simulink model "loberotator_final"  (R2018a)
settings: Solver=VariableStepAuto  StartTime=0.0  StopTime=100  RelTol=1e-3
libraries: xbsIndex_r4 x104, xps_library x4, casper_library_misc x1
(part 2 of 4)

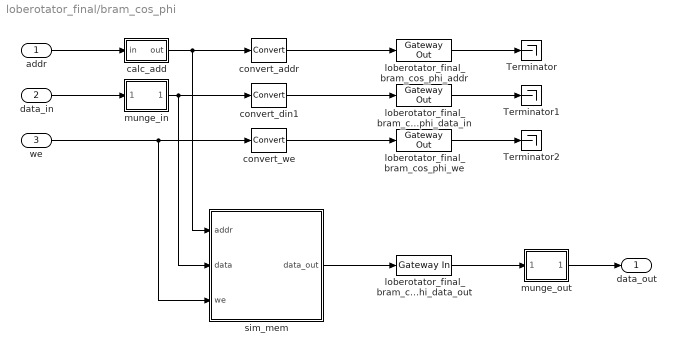
== system loberotator_final/bram_cos_phi ==
  addr : Inport
  data_in : Inport  Port=2
  we : Inport  Port=3
  Terminator : Terminator
  Terminator1 : Terminator
  Terminator2 : Terminator
  calc_add : Subsystem  mask{data_width=32, addr_width=11, sample_rate=sample_rate}
      mask prompts: data_width "data width"; addr_width "address width"; sample_rate "sample rate"
  convert_addr : xbsIndex_r4/Convert  gui_display_data_type=Fixed-point  arith_type=Unsigned  n_bits=addr_width  bin_pt=0  float_type=Single  exp_bits=8  fraction_bits=24  quantization=Truncate  overflow=Wrap  en=off  latency=0  pipeline=off  dbl_ovrd=off  block_type=convert
      settings: xl_area=[0, 0, 0, 0, 0, 0, 0]
  convert_din1 : xbsIndex_r4/Convert  gui_display_data_type=Fixed-point  arith_type=Unsigned  n_bits=32  bin_pt=0  float_type=Single  exp_bits=8  fraction_bits=24  quantization=Truncate  overflow=Wrap  en=off  latency=0  pipeline=off  dbl_ovrd=off  block_type=convert
      settings: xl_area=[0, 0, 0, 0, 0, 0, 0]
  convert_we : xbsIndex_r4/Convert  gui_display_data_type=Fixed-point  arith_type=Unsigned  n_bits=1  bin_pt=0  float_type=Single  exp_bits=8  fraction_bits=24  quantization=Truncate  overflow=Wrap  en=off  latency=0  pipeline=off  dbl_ovrd=off  block_type=convert
      settings: xl_area=[0, 0, 0, 0, 0, 0, 0]
  loberotator_final_bram_cos_phi_addr : xbsIndex_r4/Gateway Out  inherit_from_input=off  hdl_port=on  rows=1  columns=1  UseAsDAC=off  DACChannel='1'  interface=None  automatic_assignment=on  address_offset=hex2dec('00')  intf_name=''  intf_description=''  timing_constraint=None  locs_specified=off  LOCs={'A5','B9','A9','C1','A3','G6','E9','A6','A7','A8','B8','B1','B3','D9','B5','B4','B6','C2'}  io_standard={}  block_type=gatewayout
      settings: infoedit="Gateway out block.  Converts Xilinx fixed point inputs into ouputs of type Simulink integer, double, or fixed point.<P><P>Hardware notes:  In hardware these blocks become top level output ports or are discarded, depending on how they are configured."  sginterface={'Nallatech'=>{'xdspkit'=>{'non_memory_mapped_port'=>'uprev_Shared_BRAM_addr'}},'Xilinx'=>{'jtaghwcosim'=>{'non_memory_mapped_port'=>'uprev_Shared_BRAM_addr'},'xdspkit'=>{'non_memory_mapped_port'=>'uprev_Shared_BRAM_addr'}}}  xl_area=[0, 0, 0, 0, 0, 0, 0]
  loberotator_final_bram_cos_phi_data_in : xbsIndex_r4/Gateway Out  inherit_from_input=off  hdl_port=on  rows=1  columns=1  UseAsDAC=off  DACChannel='1'  interface=None  automatic_assignment=on  address_offset=hex2dec('00')  intf_name=''  intf_description=''  timing_constraint=None  locs_specified=off  LOCs={'B21','B22','A22','B23','B19','C19','A20','A21','A23','B24','A24','A25','E18','D18','C18','B18'}  io_standard={}  block_type=gatewayout
      settings: infoedit="Gateway out block.  Converts Xilinx fixed point inputs into ouputs of type Simulink integer, double, or fixed point.<P><P>Hardware notes:  In hardware these blocks become top level output ports or are discarded, depending on how they are configured."  sginterface={'Nallatech'=>{'xdspkit'=>{'non_memory_mapped_port'=>'uprev_Shared_BRAM_data_in'}},'Xilinx'=>{'jtaghwcosim'=>{'non_memory_mapped_port'=>'uprev_Shared_BRAM_data_in'},'xdspkit'=>{'non_memory_mapped_port'=>'uprev_Shared_BRAM_data_in'}}}  xl_area=[0, 0, 0, 0, 0, 0, 0]
  loberotator_final_bram_cos_phi_data_out : xbsIndex_r4/Gateway In  gui_display_data_type=Fixed-point  arith_type=Unsigned  n_bits=32  bin_pt=0  preci_type=Single  exp_width=8  frac_width=24  rows=1  columns=1  quantization=Truncate  overflow=Wrap  period=sample_rate  UseAsADC=off  ADCChannel='1'  interface=None  automatic_assignment=on  address_offset=hex2dec('00')  intf_name=''  intf_description=''  default_value=0  timing_constraint=None  locs_specified=off  LOCs={}  io_standard={}  inherit_from_input=off  hdl_port=on  dbl_ovrd=off  block_type=gatewayin
      settings: xl_area=[0, 0, 0, 0, 0, 0, 0]
  loberotator_final_bram_cos_phi_we : xbsIndex_r4/Gateway Out  inherit_from_input=off  hdl_port=on  rows=1  columns=1  UseAsDAC=off  DACChannel='1'  interface=None  automatic_assignment=on  address_offset=hex2dec('00')  intf_name=''  intf_description=''  timing_constraint=None  locs_specified=off  LOCs={'A14'}  io_standard={}  block_type=gatewayout
      settings: infoedit="Gateway out block.  Converts Xilinx fixed point inputs into ouputs of type Simulink integer, double, or fixed point.<P><P>Hardware notes:  In hardware these blocks become top level output ports or are discarded, depending on how they are configured."  xl_area=[0, 0, 0, 0, 0, 0, 0]
  munge_in : Subsystem  AncestorBlock=casper_library_flow_control/munge  mask(munge){divisions=1, div_size=32, order=[0], arith_type_out=Unsigned, bin_pt_out=0}
      mask prompts: divisions "Number of divisions"; div_size "Division size (bits)"; order "Division packing order"; arith_type_out "Output arithmetic type"; bin_pt_out "Output binary point"
      mask help: Splits an input bus into the specified number of divisions and then recombines them in the order specified (most significant division = 0,least = number divisions-1)
      mask init:
      | munge_init(gcb, ...
      |     'divisions', divisions, ...
      |     'div_size', div_size, ...
      |     'order', order, ...
      |     'arith_type_out', arith_type_out, ...
      |     'bin_pt_out', bin_pt_out);
      settings: AttributesFormatString=|
      | split:32
      | join:0
      | Unsigned [32,0]
      mask TypeOptions arith_type_out: Unsigned | Signed  (2's comp) | Floating-point
  munge_out : Subsystem  AncestorBlock=casper_library_flow_control/munge  mask(munge){divisions=1, div_size=32, order=[0], arith_type_out=Signed  (2's comp), bin_pt_out=0}
      mask prompts: divisions "Number of divisions"; div_size "Division size (bits)"; order "Division packing order"; arith_type_out "Output arithmetic type"; bin_pt_out "Output binary point"
      mask help: Splits an input bus into the specified number of divisions and then recombines them in the order specified (most significant division = 0,least = number divisions-1)
      mask init:
      | munge_init(gcb, ...
      |     'divisions', divisions, ...
      |     'div_size', div_size, ...
      |     'order', order, ...
      |     'arith_type_out', arith_type_out, ...
      |     'bin_pt_out', bin_pt_out);
      settings: AttributesFormatString=|
      | split:32
      | join:0
      | Signed  (2's comp) [32,0]
      mask TypeOptions arith_type_out: Unsigned | Signed  (2's comp) | Floating-point
  sim_mem : Subsystem  mask{arith_type=Signed  (2's comp), addr_width=11, data_width=32, data_bin_pt=0, init_vals=[2147483648      2147473531.6562      2147443182.7201      2147392601.4777      2147321788.4054      2147230744.1705      2147119469.6308      2146987965.8346      2146836234.0209      2146664275.6192      2146472092.2498      2146259685.7232      2146027058.0406      2145774211.3938       2145501148.165      2145207870.9269      2144894382.4426      2144560685.6657      2144206783.7401      2143832680.0001      2143438377.9704      2143023881.3659      2142589194.0918      2142134320.2437       2141659264.107      2141164030.1577      2140648623.0615      2140113047.6745      2139557309.0425      2138981412.4016      2138385363.1775      2137769166.9861      2137132829.6328       2136476357.113      2135799755.6116      2135103031.5033      2134386191.3524      2133649241.9127      2132892190.1272      2132115043.1288      2131317808.2393      2130500492.9699       2129663105.021      2128805652.2822      2127928142.8321       2127030584.938      2126112987.0565      2125175357.8328      2124217706.1009      2123240040.8832       2122242371.391      2121224707.0239      2120187057.3698      2119129432.2052      2118051841.4944      2116954295.3902      2115836804.2331      2114699378.5516      2113542029.0621      2112364766.6686      2111167602.4629      2109950547.7241      2108713613.9187      2107456812.7007      2106180155.9112      2104883655.5781      2103567323.9166      2102231173.3287      2100875216.4029      2099499465.9146      2098103934.8255      2096688636.2836      2095253583.6234      2093798790.3652      2092324270.2156      2090830037.0669       2089316104.997      2087782488.2697       2086229201.334      2084656258.8243      2083063675.5602      2081451466.5464      2079819646.9724      2078168232.2126      2076497237.8259      2074806679.5557      2073096573.3296      2071366935.2598      2069617781.6419      2067849128.9559      2066060993.8652       2064253393.217      2062426344.0415      2060579863.5526      2058713969.1471      2056828678.4044      2054924009.0872      2052999979.1403      2051056606.6912      2049093910.0496       2047111907.707      2045110618.3372      2043090060.7954      2041050254.1185      2038991217.5246      2036912970.4131      2034815532.3645      2032698923.1398       2030563162.681      2028408271.1101      2026234268.7298      2024041176.0225      2021829013.6507      2019597802.4564      2017347563.4611      2015078317.8656      2012790087.0499      2010482892.5727      2008156756.1713      2005811699.7617       2003447745.438      2001064915.4723      1998663232.3148       1996242718.593      1993803397.1121      1991345290.8542      1988868422.9786      1986372816.8214      1983858495.8951      1981325483.8884      1978773804.6666      1976203482.2703       1973614540.916      1971007004.9958      1968380899.0766      1965736247.9006      1963073076.3845      1960391409.6197      1957691272.8717      1954972691.5799      1952235691.3578      1949480297.9923      1946706537.4434      1943914435.8443      1941104019.5012      1938275314.8925      1935428348.6691      1932563147.6539      1929679738.8417      1926778149.3987      1923858406.6624      1920920538.1415      1917964571.5154      1914990534.6338      1911998455.5169      1908988362.3549      1905960283.5075       1902914247.504       1899850283.043      1896768418.9917      1893668684.3863      1890551108.4311      1887415720.4986      1884262550.1291      1881091627.0305      1877902981.0778      1874696642.3132      1871472640.9454      1868231007.3495      1864971772.0671       1861694965.805      1858400619.4361      1855088763.9983      1851759430.6945      1848412650.8923      1845048456.1236      1841666878.0844      1838267948.6346      1834851699.7975      1831418163.7594      1827967372.8698      1824499359.6406      1821014156.7458      1817511797.0217      1813992313.4659      1810455739.2376      1806902107.6569      1803331452.2046      1799743806.5219      1796139204.4101 ...(+39013 chars)], sample_rate=1, csp_latency=1}
      mask prompts: arith_type "Output Data Type"; addr_width "Address width"; data_width "Data width"; data_bin_pt "Data Binary Point"; init_vals "Initial values"; sample_rate "Sample rate"; csp_latency "Latency"
      mask init:
      | % set_param([gcb, '/data_to_xilinx'], 'arith_type', arith_type)
      | % set_param([gcb, '/data_to_xilinx'], 'n_bits', get_param(gcb, 'data_width'))
      mask TypeOptions arith_type: Unsigned | Signed  (2's comp)
      mask TypeOptions data_width: 8 | 16 | 32 | 64 | 128
  data_out : Outport
  wires:
  munge_out/1(dout) -> data_out/1
  sim_mem/1(data_out) -> loberotator_final_bram_cos_phi_data_out/1
  loberotator_final_bram_cos_phi_data_out/1 -> munge_out/1(din)
  convert_addr/1 -> loberotator_final_bram_cos_phi_addr/1
  convert_din1/1 -> loberotator_final_bram_cos_phi_data_in/1
  data_in/1 -> munge_in/1(din)
  calc_add/1(out) -> sim_mem/1(addr), convert_addr/1
  loberotator_final_bram_cos_phi_we/1 -> Terminator2/1
  loberotator_final_bram_cos_phi_data_in/1 -> Terminator1/1
  loberotator_final_bram_cos_phi_addr/1 -> Terminator/1
  convert_we/1 -> loberotator_final_bram_cos_phi_we/1
  addr/1 -> calc_add/1(in)
  we/1 -> sim_mem/3(we), convert_we/1
  munge_in/1(dout) -> sim_mem/2(data), convert_din1/1
